simulink model "Clock"  (R2017b)
settings: Solver=FixedStepDiscrete  StartTime=0.0  StopTime=20  FixedStep=0.200000  RelTol=1e-3
model workspace (MAT data in the model file):
  input_struct.time = [0; 0.2; 0.4; 0.6; 0.8; 1; 1.2; 1.4; 1.6; 1.8; 2; 2.2; 2.4; 2.6; 2.8; 3; 3.2; 3.4; 3.6; 3.8; 4; 4.2; 4.4; 4.6; 4.8; 5; 5.2; 5.4; 5.6; 5.8; 6; 6.2; 6.4; 6.6; 6.8; 7; 7.2; 7.4; 7.6; 7.8; 8; 8.2; 8.4; 8.6; 8.8; 9; 9.2; 9.4; 9.6; 9.8; 10; 10.2; 10.4; 10.6; 10.8; 11; 11.2; 11.4; 11.6; 11.8; 12; 12.2; 12.4; 12.6; 12.8; 13; 13.2; 13.4; 13.6; 13.8; 14; 14.2; 14.4; 14.6; 14.8; 15; 15.2; 15.4; 15.6; 15.8; 16; 16.2; 16.4; 16.6; 16.8; 17; 17.2; 17.4; 17.6; 17.8; 18; 18.2; 18.4; 18.6; 18.8; 19; 19.2; 19.4; 19.6; 19.8]
  input_struct.signals.name = 'In1'
  input_struct.signals.values = [22.0807238781; -82.2074741714; -26.6389025255; 87.9904849925; 84.5627025133; -47.8285422916; -47.0853416894; 56.066159441; -19.6184416781; 77.2911833251; -9.56258720468; -0.602294653453; -25.4076267862; -23.6580916183; -8.38286981738; 43.556989153; 45.9902536991; -32.7735873675; -7.14041079254; -24.4588574767; -87.2100350385; 96.5403907535; 19.2586364379; -9.97263319999; 94.4021177195; 37.7308787354; -2.4033262527; -28.5307078317; -13.7024109637; -58.7610458591; 8.96998189594; 91.5004175055; -62.5989660662; 54.0409590676; 67.4761002089; 81.6627480711; 26.1326141353; 18.718889785; 54.5205288575; -45.3862702758; -98.3524769914; -46.3162390601; 6.77092783873; -54.971773706; 82.4982023837; -77.4522917934; -46.7315913579; -4.04078648086; 32.186864581; 67.1894182623; 26.9425460611; 61.368123389; 14.4840672819; -1.65773861738; 60.3027334634; -11.7897199006; -90.2260545629; 97.4920581812; 49.849895669; 15.7289543675; -33.1666823456; 18.6703985836; 80.3288583967; 68.5890280636; 73.6832267842; -79.2725603203; 57.4621218993; -18.8078210695; -38.6066308638; -94.6959350847; 42.0911751291; 68.725513913; -90.0224389436; -50.873719389; 90.0313627611; -77.9839231799; 91.5949976544; -30.9227932685; 76.0896392314; -44.794098502; 42.8897073321; -90.0568510502; -78.5492875688; 71.798150706; -15.1441063776; 12.5051370011; 46.544918861; 92.1765964922; -88.173003222; -76.086782397; -73.8399696727; 60.5441031033; -67.9658285663; 5.10605089644; 41.7184305835; 98.0792401049; 22.0870338603; -41.6835405363; 10.1760327201; 8.14211799825]
  input_struct.signals.dimensions = 1
settings Model: Creator=hbourbou  LastModifiedBy=hbourbou
settings SolverCC: InsertRTBMode=Never (minimum delay)
settings DataIOCC: ExternalInput=input_struct  LimitDataPoints=on  LoadExternalInput=on  SaveFormat=Array
settings OptimizationCC: LifeSpan=inf
settings DebuggingCC: SFUnexpectedBacktrackingDiag=warning  SFNoUnconditionalDefaultTransitionDiag=warning  SFExecutionAtInitializationDiag=none
settings HardwareCC: ProdBitPerPointer=32  ProdBitPerSizeT=32  ProdBitPerPtrDiffT=32  ProdLargestAtomicFloat=None  ProdIntDivRoundTo=Undefined  ProdEndianess=Unspecified  ProdWordSize=32  ProdHWDeviceType=32-bit Generic
settings ModelReferenceCC: PropagateSignalLabelsOutOfModel=off
settings CodeAppCC: StateflowObjectComments=on
settings GRTTargetCC: TargetLangStandard=C89/C90 (ANSI)  GeneratePreprocessorConditionals=Disable all
settings ConfigComp: CovMetricSettings=dw  CovHtmlReporting=on  CovSaveCumulativeToWorkspaceVar=on  CovSaveSingleToWorkspaceVar=on  CovExternalEMLEnable=off

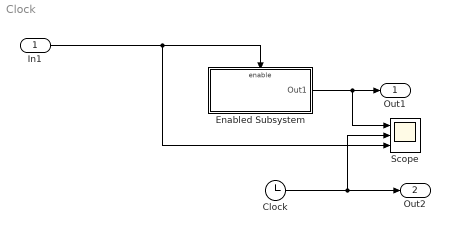
== system Clock ==
  In1 : Inport
  Clock : Clock
  Enabled Subsystem : Subsystem  TreatAsAtomicUnit=on
  Scope : Scope  NumInputPorts=3
  Out1 : Outport
  Out2 : Outport  Port=2
  wires:
  In1/1 -> Scope/3, Enabled Subsystem/Enable
  Enabled Subsystem/1(Out1) -> Scope/1, Out1/1
  Clock/1 -> Scope/2, Out2/1

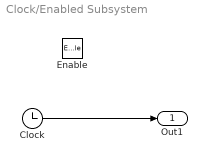
== system Clock/Enabled Subsystem ==
  Enable : EnablePort  StatesWhenEnabling=reset
  Clock : Clock
  Out1 : Outport
  wires:
  Clock/1 -> Out1/1
